simulink model "model"  (R2015a)
settings: Solver=ode45  StartTime=0.0  StopTime=2  RelTol=1e-3
settings Model: Creator=admin  LastModifiedBy=admin

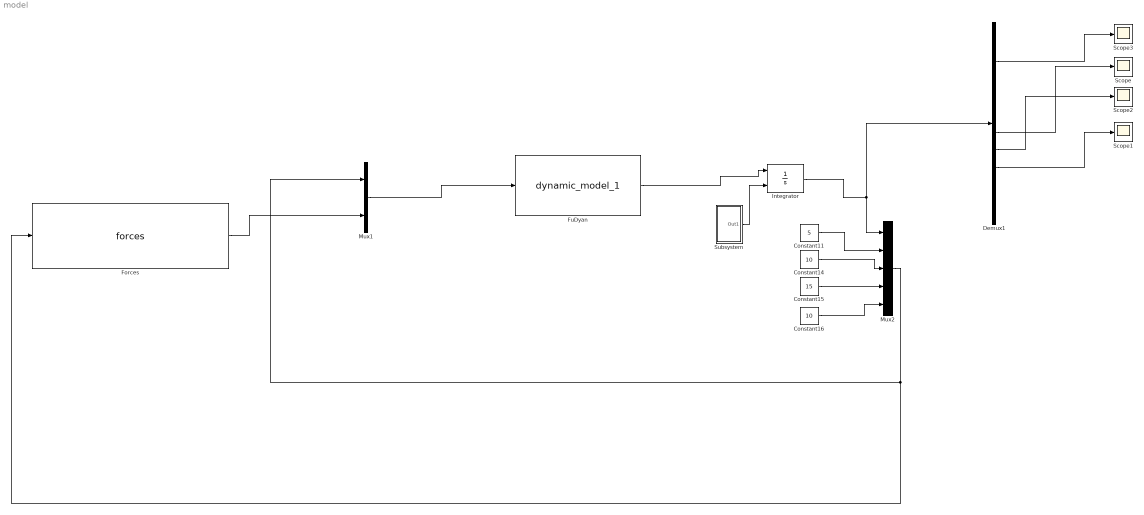
== system model ==
  " FuDyan" : MATLABFcn  MATLABFcn=dynamic_model_1
  Constant11 : Constant  Value=5
  Constant14 : Constant  Value=10
  Constant15 : Constant  Value=15
  Constant16 : Constant  Value=10
  Demux1 : Demux  Outputs=12
  Forces : MATLABFcn  MATLABFcn=forces  OutputDimensions=24
  Integrator : Integrator  InitialConditionSource=external
  Mux1 : Mux  Inputs=2
  Mux2 : Mux  Inputs=5
  Scope{,1..3} (4 alike) : Scope
      Scope2 settings: SaveName=ScopeData2
      Scope3 settings: SaveName=ScopeData3
  Subsystem : Subsystem
  wires:
  " FuDyan"/1 -> Integrator/1
  Mux2/1 -> Mux1/1, Forces/1
  Integrator/1 -> Demux1/1, Mux2/1
  Constant11/1 -> Mux2/2
  Constant14/1 -> Mux2/3
  Constant15/1 -> Mux2/4
  Constant16/1 -> Mux2/5
  Mux1/1 -> " FuDyan"/1
  Forces/1 -> Mux1/2
  Subsystem/1(Out1) -> Integrator/2
  Demux1/7 -> Scope/1
  Demux1/8 -> Scope2/1
  Demux1/9 -> Scope1/1
  Demux1/3 -> Scope3/1

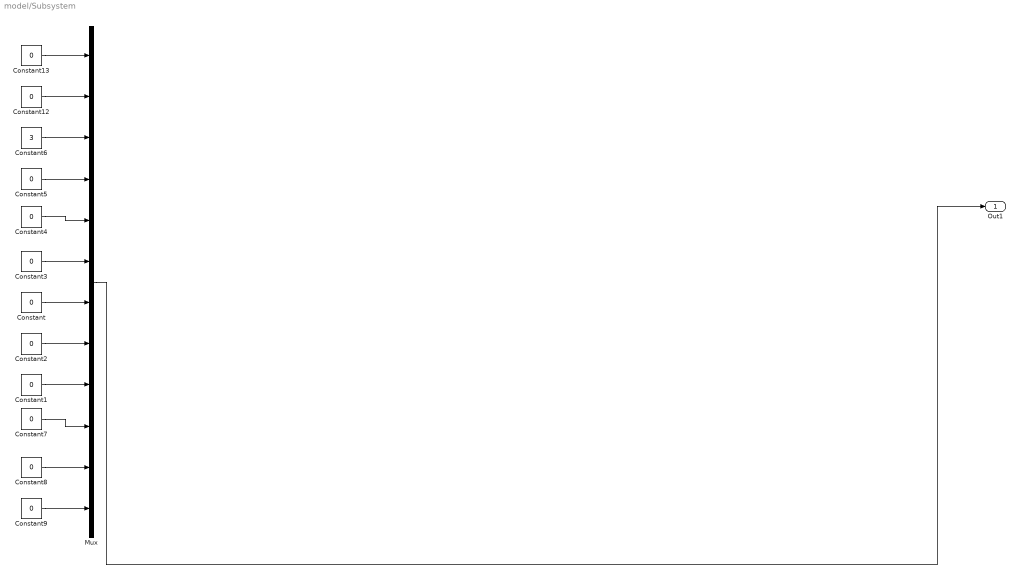
== system model/Subsystem ==
  Constant{,1..5,7..9,12..13} (11 alike) : Constant  Value=0
  Constant6 : Constant  Value=3
  Mux : Mux  Inputs=12
  Out1 : Outport
  wires:
  Constant/1 -> Mux/7
  Constant13/1 -> Mux/1
  Mux/1 -> Out1/1
  Constant2/1 -> Mux/8
  Constant4/1 -> Mux/5
  Constant9/1 -> Mux/12
  Constant3/1 -> Mux/6
  Constant5/1 -> Mux/4
  Constant8/1 -> Mux/11
  Constant1/1 -> Mux/9
  Constant12/1 -> Mux/2
  Constant6/1 -> Mux/3
  Constant7/1 -> Mux/10
